simulink model "Trayectoria"  (R2023b)
settings: Solver=ode8  StartTime=0.0  StopTime=t6  FixedStep=0.01  RelTol=1e-3
undefined symbols (not defined in the file): alpha8, cL, cO, cpL, cpO, cpS, cS, gammaO, gammaS, k1, k2, k3, k4, klL, klO, klS, muO, muS, r8, t3, xr8, xrLB, xrLH, xrLPA, xrLR, xrLSA, xrLTA, xrO, xrS
libraries: vrlib x1
settings Model: Creator=olegalexandrocraviotog.  LastModifiedBy=olegalexandrocraviotog.

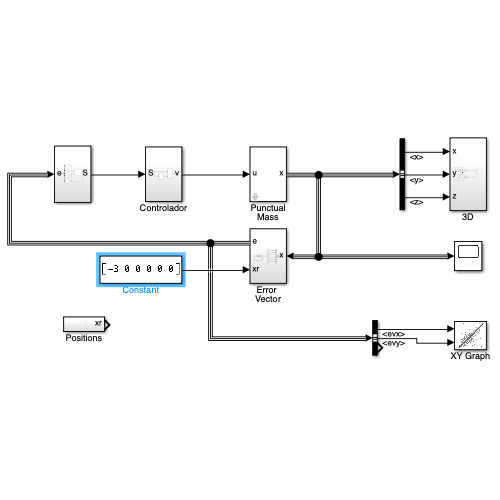
[thumbnail: Simulink's stored preview of the top-level diagram]
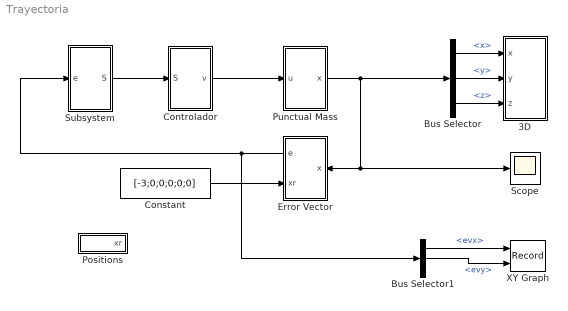
== system Trayectoria ==
  3D : Subsystem
  Bus Selector : BusSelector  OutputSignals=x,y,z
  Bus Selector1 : BusSelector  OutputSignals=evx,evy,evz
  Constant : Constant  Value=[-3;0;0;0;0;0]
  Controlador : Subsystem
  Error Vector : Subsystem
      settings: PortSchema="{\"entries\":[{\"content\":{\"sides\":[{\"content\":{\"connectorIds\":[\"Out1\",\"In1\"]},\"type\":\"ConnectorPlacement.EquallySpacedRectSide\",\"uuid\":\"f657f758-fbd3-4a41-9063-d27a9332990f\"},{\"content\":{\"connectorIds\":[\"In2\"],\"side\":\"RIGHT\"},\"type\":\"ConnectorPlacement.EquallySpacedRectSide\",\"uuid\":\"1c515ff8-89aa-408f-b30d-a9af781c1d92\"},{\"content\":{\"side\":\"TOP\"},\"type\":\"ConnectorPlacement.EquallySpacedRectSide\",\"uuid\":\"e6b04dad-d129-4308-a4a4-85eae89abd10\"}]},\"type\":\"ConnectorPlacement.EquallySpacedConnector\",\"uuid\":\"97b78294-1485-42d0-98d9-31abf3c44744\"}],\"packageUris\":[\"http://schema.mathworks.com/mf0/Connector/R2020b\"],\"version\":\"1.0\"}"
  Positions : Subsystem
  Punctual Mass : Subsystem  mask{A=[0 0 0 1 0 0; 0 0 0 0 1 0; 0 0 0 0 0 1; 0 0 0 0 0 0; 0 0 0 0 0 0; 0 0 0 0 0 0], B=[0 0 0; 0 0 0; 0 0 0; 1 0 0; 0 1 0; 0 0 1]}
  Scope : Scope
  Subsystem : Subsystem
  XY Graph : Record  FileSettingsInternal="{\"entries\":[{\"content\":{\"excelSettings\":{\"content\":{},\"type\":\"Streamout.ExcelSettings\"}},\"type\":\"Streamout.FileSettingStorage\",\"uuid\":\"\"}],\"packageUris\":[\"http:\\/\\/schema.mathworks.com\\/mf0\\/streamout_blocks\\/R2020a\"],\"version\":\"1.0\"}"  Layout=[1 1]  SignalsInternal="{\"entries\":[{\"content\":{\"signals\":[{\"content\":{\"blockPath\":[],\"dimensions\":[1],\"domain\":\"\",\"lineColor\":\"#a2142f\",\"plots\":[1],\"port\":1,\"sid\":[\"\"],\"signalID\":12236,\"signalName\":\"<evx>\"},\"type\":\"RecordBlkView.Signal\",\"uuid\":\"\"},{\"content\":{\"blockPath\":[],\"dimensions\":[1],\"domain\":\"\",\"lineColor\":\"#139fff\",\"plots\":[1],\"port\":2,\"sid\":[\"\"],\"signalID\":12240,\"signalName\":\"<evy>\"},\"type\":\"RecordBlkView.Signal\",\"uuid\":\"\"}]},\"type\":\"RecordBlkView.InputSignals\",\"uuid\":\"\"}],\"packageUris\":[\"http:\\/\\/schema.mathworks.com\\/mf0\\/streamout_blocks\\/R2020a\"],\"version\":\"1.0\"}"  VisualizationBindings="{\"xyplotplugin\":{\"info\":[{\"series\":[{\"bindingParametersList\":[{\"parameter\":\"X-Axis\",\"signalID\":12236,\"signalName\":\"<evx>\"},{\"parameter\":\"Y-Axis\",\"signalID\":12240,\"signalName\":\"<evy>\"}],\"seriesID\":43551}],\"subplotID\":1}]}}"  CompatibilityTag=XY
  wires:
  Punctual Mass/1(x) -> Scope/1, Error Vector/2(x), Bus Selector/1
  Bus Selector/1 -> 3D/1(x)  "<x>"
  Bus Selector/2 -> 3D/2(y)  "<y>"
  Bus Selector/3 -> 3D/3(z)  "<z>"
  Controlador/1(v) -> Punctual Mass/1(u)
  Subsystem/1(S) -> Controlador/1(S)
  Error Vector/1(e) -> Subsystem/1(e), Bus Selector1/1
  Bus Selector1/1 -> XY Graph/1  "<evx>"
  Constant/1 -> Error Vector/1(xr)
  Bus Selector1/2 -> XY Graph/2  "<evy>"

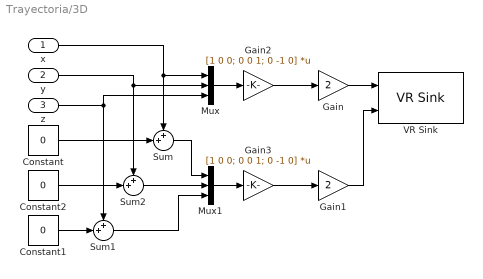
== system Trayectoria/3D ==
  x : Inport
  y : Inport  Port=2
  z : Inport  Port=3
  Constant : Constant  Value=0
  Constant1 : Constant  Value=0
  Constant2 : Constant  Value=0
  Gain : Gain  Gain=2
  Gain1 : Gain  Gain=2
  Gain2 : Gain  Gain=[1 0 0; 0 0 1; 0 -1 0]  Multiplication=Matrix(K*u)
  Gain3 : Gain  Gain=[1 0 0; 0 0 1; 0 -1 0]  Multiplication=Matrix(K*u)
  Mux : Mux  Inputs=3
  Mux1 : Mux  Inputs=3
  Sum : Sum  Inputs=++|
  Sum1 : Sum  Inputs=++|
  Sum2 : Sum  Inputs=++|
  VR Sink : vrlib/VR Sink  InstantiateOnLoad=on  SampleTime=0.01  ViewEnable=on  RemoteChange=off  RemoteView=off  FieldsWritten=Masa.translation.3.1.1.double#Pelota.position.3.1.1.double  WorldFileName=/Users/olegalexandrocraviotog./Documents/MATLAB/MasaPuntual/Imagenes3D/Trayectoria3D.x3d  AutoView=off  VideoDimensions=[]  AllowVariableSize=off
  wires:
  z/1 -> Sum1/1, Mux/3
  y/1 -> Sum2/1, Mux/2
  x/1 -> Mux/1, Sum/1
  Gain2/1 -> Gain/1
  Mux/1 -> Gain2/1
  Sum1/1 -> Mux1/3
  Sum2/1 -> Mux1/2
  Sum/1 -> Mux1/1
  Gain3/1 -> Gain1/1
  Constant2/1 -> Sum2/2
  Constant1/1 -> Sum1/2
  Gain1/1 -> VR Sink/2
  Constant/1 -> Sum/2
  Mux1/1 -> Gain3/1
  Gain/1 -> VR Sink/1

== system Trayectoria/Controlador ==
  S : Inport
  Subsystem1 : Subsystem
  Subsystem2 : Subsystem
  v : Outport
  wires:
  S/1 -> Subsystem2/1(S), Subsystem1/1(S)
  Subsystem2/1(dZ) -> Subsystem1/2(dZ)
  Subsystem1/1(v) -> v/1

== system Trayectoria/Error Vector ==
  xr : Inport
  x : Inport  Port=2
  Bus Creator : BusCreator  Inputs=6
  Demux : Demux  Outputs=6
  Sum : Sum  Inputs=|+-
  e : Outport
  wires:
  x/1 -> Sum/1
  xr/1 -> Sum/2
  Bus Creator/1 -> e/1
  Sum/1 -> Demux/1
  Demux/1 -> Bus Creator/1  "ex"
  Demux/2 -> Bus Creator/2  "ey"
  Demux/3 -> Bus Creator/3  "ez"
  Demux/4 -> Bus Creator/4  "evx"
  Demux/5 -> Bus Creator/5  "evy"
  Demux/6 -> Bus Creator/6  "evz"

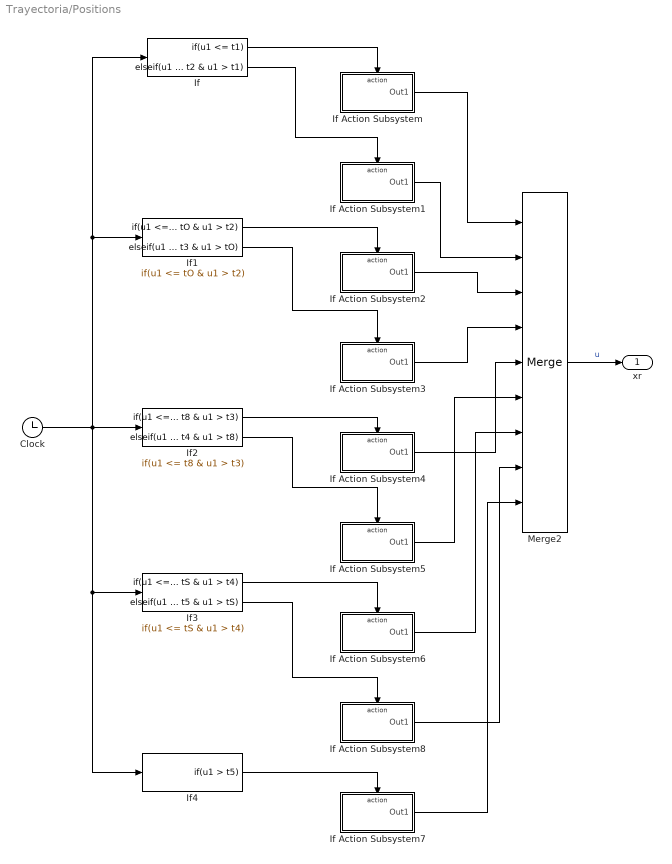
== system Trayectoria/Positions ==
  Clock : Clock
  If : If  IfExpression=u1 <= t1  ElseIfExpressions=u1 <= t2 & u1 > t1  ShowElse=off
  If Action Subsystem : Subsystem  TreatAsAtomicUnit=on
  If Action Subsystem1 : Subsystem  TreatAsAtomicUnit=on
  If Action Subsystem2 : Subsystem  TreatAsAtomicUnit=on
  If Action Subsystem3 : Subsystem  TreatAsAtomicUnit=on
  If Action Subsystem4 : Subsystem  TreatAsAtomicUnit=on
  If Action Subsystem5 : Subsystem  TreatAsAtomicUnit=on
  If Action Subsystem6 : Subsystem  TreatAsAtomicUnit=on
  If Action Subsystem7 : Subsystem  TreatAsAtomicUnit=on
  If Action Subsystem8 : Subsystem  TreatAsAtomicUnit=on
  If1 : If  IfExpression=u1 <= tO & u1 > t2  ElseIfExpressions=u1 <= t3 & u1 > tO  ShowElse=off
  If2 : If  IfExpression=u1 <= t8 & u1 > t3  ElseIfExpressions=u1 <= t4 & u1 > t8  ShowElse=off
  If3 : If  IfExpression=u1 <= tS & u1 > t4  ElseIfExpressions=u1 <= t5 & u1 > tS  ShowElse=off
  If4 : If  IfExpression=u1 > t5  ShowElse=off
  Merge2 : Merge  Inputs=9
  xr : Outport
  wires:
  If/1 -> If Action Subsystem/Action
  Clock/1 -> If3/1, If4/1, If2/1, If1/1, If/1
  Merge2/1 -> xr/1  "u"
  If Action Subsystem/1(Out1) -> Merge2/1
  If Action Subsystem1/1(Out1) -> Merge2/2
  If Action Subsystem2/1(Out1) -> Merge2/3
  If Action Subsystem3/1(Out1) -> Merge2/4
  If Action Subsystem4/1(Out1) -> Merge2/5
  If Action Subsystem5/1(Out1) -> Merge2/6
  If Action Subsystem6/1(Out1) -> Merge2/7
  If Action Subsystem8/1(Out1) -> Merge2/8
  If Action Subsystem7/1(Out1) -> Merge2/9
  If/2 -> If Action Subsystem1/Action
  If1/1 -> If Action Subsystem2/Action
  If1/2 -> If Action Subsystem3/Action
  If2/1 -> If Action Subsystem4/Action
  If2/2 -> If Action Subsystem5/Action
  If3/1 -> If Action Subsystem6/Action
  If3/2 -> If Action Subsystem8/Action
  If4/1 -> If Action Subsystem7/Action

== system Trayectoria/Punctual Mass ==
  u : Inport
  Bus Creator : BusCreator  Inputs=6
  Constant : Constant  Value=[0;0;0]
  Demux : Demux  Outputs=6
  Gain : Gain  Gain=A  Multiplication=Matrix(K*u)
  Gain1 : Gain  Gain=B  Multiplication=Matrix(K*u)
  Integrator : Integrator  InitialCondition=[0;0;0;0;0;0]
  Sum : Sum  Inputs=|++
  Sum1 : Sum  Inputs=++|
  x : Outport
  wires:
  u/1 -> Sum1/2
  Sum1/1 -> Gain1/1
  Constant/1 -> Sum1/1
  Gain1/1 -> Sum/1
  Integrator/1 -> Gain/1, Demux/1
  Sum/1 -> Integrator/1
  Gain/1 -> Sum/2
  Demux/3 -> Bus Creator/3  "z"
  Demux/1 -> Bus Creator/1  "x"
  Demux/2 -> Bus Creator/2  "y"
  Demux/4 -> Bus Creator/4  "vx"
  Demux/5 -> Bus Creator/5  "vy"
  Demux/6 -> Bus Creator/6  "vz"
  Bus Creator/1 -> x/1

== system Trayectoria/Subsystem ==
  e : Inport
  Descendent Spiral : Subsystem
  Eight on a Sphere : Subsystem
  Looping : Subsystem
  Positions : Subsystem
  Staight Line : Subsystem
  S : Outport
  wires:
  e/1 -> Looping/1(e), Staight Line/1(e), Descendent Spiral/1(e), Eight on a Sphere/1(e)
  Staight Line/1(Sj) -> Positions/1(Straight Line)
  Eight on a Sphere/1(S4) -> Positions/3(Egith on a Sphere)
  Descendent Spiral/1(S6) -> Positions/4(Descending Spiral), S/1
  Looping/1(S6) -> Positions/2(Looping)

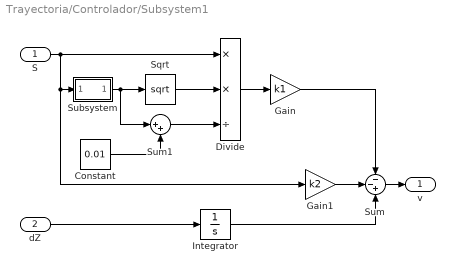
== system Trayectoria/Controlador/Subsystem1 ==
  S : Inport
  dZ : Inport  Port=2
  Constant : Constant  Value=0.01
  Divide : Product  Inputs=**/
  Gain : Gain  Gain=k1
  Gain1 : Gain  Gain=k2
  Integrator : Integrator
  Sqrt : Sqrt
  Subsystem : Subsystem
      mask Display: disp('||  ||');
  Sum : Sum  Inputs=--+
  Sum1 : Sum  Inputs=|++
  v : Outport
  wires:
  dZ/1 -> Integrator/1
  Divide/1 -> Gain/1
  Sum1/1 -> Divide/3
  Sum/1 -> v/1
  Integrator/1 -> Sum/3
  S/1 -> Gain1/1, Subsystem/1(In1), Divide/1
  Subsystem/1(Out1) -> Sum1/1, Sqrt/1
  Constant/1 -> Sum1/2
  Gain1/1 -> Sum/2
  Sqrt/1 -> Divide/2
  Gain/1 -> Sum/1

== system Trayectoria/Controlador/Subsystem2 ==
  S : Inport
  Constant : Constant  Value=0.01
  Gain2 : Gain  Gain=k3
  Gain3 : Gain  Gain=k4
  Product : Product  Inputs=*/
  Subsystem : Subsystem
      mask Display: disp('||  ||');
  Sum : Sum  Inputs=|++
  Sum1 : Sum  Inputs=--
  dZ : Outport
  wires:
  Sum1/1 -> dZ/1
  Subsystem/1(Out1) -> Sum/1
  Product/1 -> Gain2/1
  Gain3/1 -> Sum1/2
  Sum/1 -> Product/2
  Constant/1 -> Sum/2
  Gain2/1 -> Sum1/1
  S/1 -> Product/1, Gain3/1, Subsystem/1(In1)

== system Trayectoria/Positions/If Action Subsystem ==
  Action Port : ActionPort  ActionPortLabel=if(u1 <= t1)
  Constant : Constant  Value=xrLH
  Out1 : Outport
  wires:
  Constant/1 -> Out1/1

== system Trayectoria/Positions/If Action Subsystem1 ==
  Action Port : ActionPort  ActionPortLabel=elseif(u1 <= t2 & u1 > t1)
  Constant : Constant  Value=xrLPA
  Out1 : Outport
  wires:
  Constant/1 -> Out1/1

== system Trayectoria/Positions/If Action Subsystem2 ==
  Action Port : ActionPort  ActionPortLabel=if(u1 <= tO & u1 > t2)
  Constant : Constant  Value=xrO
  Out1 : Outport
  wires:
  Constant/1 -> Out1/1

== system Trayectoria/Positions/If Action Subsystem3 ==
  Action Port : ActionPort  ActionPortLabel=elseif(u1 <= t3 & u1 > tO)
  Constant : Constant  Value=xrLSA
  Out1 : Outport
  wires:
  Constant/1 -> Out1/1

== system Trayectoria/Positions/If Action Subsystem4 ==
  Action Port : ActionPort  ActionPortLabel=if(u1 <= t8 & u1 > t3)
  Constant : Constant  Value=xr8
  Out1 : Outport
  wires:
  Constant/1 -> Out1/1

== system Trayectoria/Positions/If Action Subsystem5 ==
  Action Port : ActionPort  ActionPortLabel=elseif(u1 <= t4 & u1 > t8)
  Constant : Constant  Value=xrLTA
  Out1 : Outport
  wires:
  Constant/1 -> Out1/1

== system Trayectoria/Positions/If Action Subsystem6 ==
  Action Port : ActionPort  ActionPortLabel=if(u1 <= tS & u1 > t4)
  Constant : Constant  Value=xrS
  Out1 : Outport
  wires:
  Constant/1 -> Out1/1

== system Trayectoria/Positions/If Action Subsystem7 ==
  Action Port : ActionPort  ActionPortLabel=if(u1 > t5)
  Constant : Constant  Value=xrLB
  Out1 : Outport
  wires:
  Constant/1 -> Out1/1

== system Trayectoria/Positions/If Action Subsystem8 ==
  Action Port : ActionPort  ActionPortLabel=elseif(u1 <= t5 & u1 > tS)
  Constant : Constant  Value=xrLR
  Out1 : Outport
  wires:
  Constant/1 -> Out1/1

== system Trayectoria/Subsystem/Descendent Spiral ==
  e : Inport
  Bus Selector3 : BusSelector  OutputSignals=ez,evz
  Mux : Mux  Inputs=3
  Subsystem : Subsystem  mask{mu=muS, gama=gammaS}
      mask prompts: gama "gamma"
  Subsystem1 : Subsystem  mask{mu=muS, gama=gammaS}
      mask prompts: gama "gamma"
  Subsystem2 : Subsystem  mask{k=klS, c=cS, cp=cpS}
  S6 : Outport
  wires:
  Mux/1 -> S6/1
  Subsystem2/1(Sz) -> Mux/3
  Bus Selector3/2 -> Subsystem2/2(ev)  "<evz>"
  Bus Selector3/1 -> Subsystem2/1(e)  "<ez>"
  e/1 -> Subsystem1/1(e), Subsystem/1(e), Bus Selector3/1
  Subsystem1/1(Sy) -> Mux/2
  Subsystem/1(Sx) -> Mux/1

== system Trayectoria/Subsystem/Eight on a Sphere ==
  e : Inport
  Mux : Mux  Inputs=3
  Subsystem : Subsystem  mask{apha=alpha8, r=r8}
      mask prompts: apha "alpha"
  Subsystem1 : Subsystem  mask{apha=alpha8, r=r8}
      mask prompts: apha "alpha"
  Subsystem2 : Subsystem  mask{apha=alpha8, r=r8}
      mask prompts: apha "alpha"
  S4 : Outport
  wires:
  e/1 -> Subsystem2/1(e), Subsystem/1(e), Subsystem1/1(e)
  Subsystem1/1(Sy) -> Mux/2
  Subsystem/1(Sx) -> Mux/1
  Subsystem2/1(Sz) -> Mux/3
  Mux/1 -> S4/1

== system Trayectoria/Subsystem/Looping ==
  e : Inport
  Bus Selector3 : BusSelector  OutputSignals=ey,evy
  Mux : Mux  Inputs=3
  Subsystem : Subsystem  mask{mu=muO, gama=gammaO}
      mask prompts: gama "gamma"
  Subsystem1 : Subsystem  mask{mu=muO, gama=gammaO}
      mask prompts: gama "gamma"
  Subsystem2 : Subsystem  mask{k=klO, c=cO, cp=cpO}
  S6 : Outport
  wires:
  Subsystem/1(Sx) -> Mux/1
  e/1 -> Bus Selector3/1, Subsystem/1(e), Subsystem1/1(e)
  Bus Selector3/1 -> Subsystem2/1(e)  "<ey>"
  Bus Selector3/2 -> Subsystem2/2(ev)  "<evy>"
  Mux/1 -> S6/1
  Subsystem2/1(Sy) -> Mux/2
  Subsystem1/1(Sz) -> Mux/3

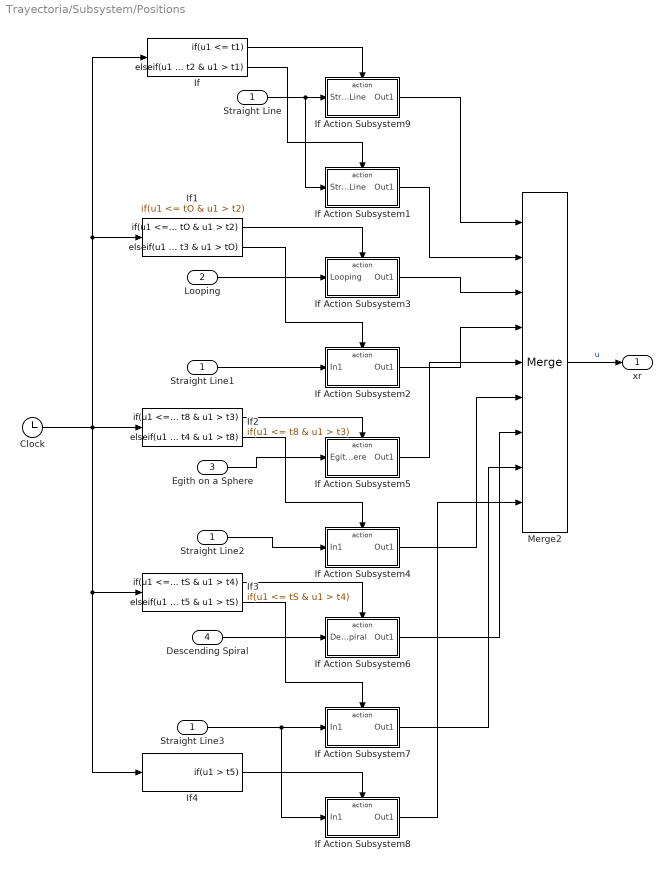
== system Trayectoria/Subsystem/Positions ==
  Straight Line : Inport
  Looping : Inport  Port=2
  Egith on a Sphere : Inport  Port=3
  Descending Spiral : Inport  Port=4
  Clock : Clock
  If : If  IfExpression=u1 <= t1  ElseIfExpressions=u1 <= t2 & u1 > t1  ShowElse=off
  If Action Subsystem1 : Subsystem  TreatAsAtomicUnit=on
  If Action Subsystem2 : Subsystem  TreatAsAtomicUnit=on
  If Action Subsystem3 : Subsystem  TreatAsAtomicUnit=on
  If Action Subsystem4 : Subsystem  TreatAsAtomicUnit=on
  If Action Subsystem5 : Subsystem  TreatAsAtomicUnit=on
  If Action Subsystem6 : Subsystem  TreatAsAtomicUnit=on
  If Action Subsystem7 : Subsystem  TreatAsAtomicUnit=on
  If Action Subsystem8 : Subsystem  TreatAsAtomicUnit=on
  If Action Subsystem9 : Subsystem  TreatAsAtomicUnit=on
  If1 : If  IfExpression=u1 <= tO & u1 > t2  ElseIfExpressions=u1 <= t3 & u1 > tO  ShowElse=off
  If2 : If  IfExpression=u1 <= t8 & u1 > t3  ElseIfExpressions=u1 <= t4 & u1 > t8  ShowElse=off
  If3 : If  IfExpression=u1 <= tS & u1 > t4  ElseIfExpressions=u1 <= t5 & u1 > tS  ShowElse=off
  If4 : If  IfExpression=u1 > t5  ShowElse=off
  Merge2 : Merge  Inputs=9
  Straight Line1 : InportShadow
  Straight Line2 : InportShadow
  Straight Line3 : InportShadow
  xr : Outport
  wires:
  Clock/1 -> If3/1, If4/1, If2/1, If1/1, If/1
  Merge2/1 -> xr/1  "u"
  If/1 -> If Action Subsystem9/Action
  If/2 -> If Action Subsystem1/Action
  If1/1 -> If Action Subsystem3/Action
  If1/2 -> If Action Subsystem2/Action
  If2/1 -> If Action Subsystem5/Action
  If2/2 -> If Action Subsystem4/Action
  If3/1 -> If Action Subsystem6/Action
  If3/2 -> If Action Subsystem7/Action
  If4/1 -> If Action Subsystem8/Action
  Straight Line/1 -> If Action Subsystem1/1(Straight Line), If Action Subsystem9/1(Straight Line)
  Looping/1 -> If Action Subsystem3/1(Looping)
  Straight Line1/1 -> If Action Subsystem2/1(In1)
  Egith on a Sphere/1 -> If Action Subsystem5/1(Egith on a Sphere)
  Straight Line2/1 -> If Action Subsystem4/1(In1)
  Descending Spiral/1 -> If Action Subsystem6/1(Descending Spiral)
  Straight Line3/1 -> If Action Subsystem8/1(In1), If Action Subsystem7/1(In1)
  If Action Subsystem9/1(Out1) -> Merge2/1
  If Action Subsystem1/1(Out1) -> Merge2/2
  If Action Subsystem3/1(Out1) -> Merge2/3
  If Action Subsystem2/1(Out1) -> Merge2/4
  If Action Subsystem5/1(Out1) -> Merge2/5
  If Action Subsystem4/1(Out1) -> Merge2/6
  If Action Subsystem6/1(Out1) -> Merge2/7
  If Action Subsystem7/1(Out1) -> Merge2/8
  If Action Subsystem8/1(Out1) -> Merge2/9

== system Trayectoria/Subsystem/Staight Line ==
  e : Inport
  Bus Selector1 : BusSelector  OutputSignals=ex,evx
  Bus Selector2 : BusSelector  OutputSignals=ey,evy
  Bus Selector3 : BusSelector  OutputSignals=ez,evz
  Mux : Mux  Inputs=3
  Subsystem : Subsystem  mask{k=klL(1), c=cL(1), cp=cpL(1)}
  Subsystem1 : Subsystem  mask{k=klL(2), c=cL(2), cp=cpL(2)}
  Subsystem2 : Subsystem  mask{k=klL(3), c=cL(3), cp=cpL(3)}
  Sj : Outport
  wires:
  e/1 -> Bus Selector1/1, Bus Selector3/1, Bus Selector2/1
  Bus Selector1/1 -> Subsystem/1(e)  "<ex>"
  Bus Selector1/2 -> Subsystem/2(ev)  "<evx>"
  Bus Selector2/1 -> Subsystem1/1(e)  "<ey>"
  Bus Selector2/2 -> Subsystem1/2(ev)  "<evy>"
  Bus Selector3/1 -> Subsystem2/1(e)  "<ez>"
  Bus Selector3/2 -> Subsystem2/2(ev)  "<evz>"
  Subsystem1/1(Sy) -> Mux/2
  Subsystem/1(Sx) -> Mux/1
  Subsystem2/1(Sz) -> Mux/3
  Mux/1 -> Sj/1

== system Trayectoria/Controlador/Subsystem1/Subsystem ==
  In1 : Inport
  Dot Product : DotProduct  OutDataTypeStr=Inherit: Inherit via internal rule
  Sqrt : Sqrt
  Out1 : Outport
  wires:
  Dot Product/1 -> Sqrt/1
  Sqrt/1 -> Out1/1
  In1/1 -> Dot Product/2, Dot Product/1

== system Trayectoria/Controlador/Subsystem2/Subsystem ==
  In1 : Inport
  Dot Product : DotProduct  OutDataTypeStr=Inherit: Inherit via internal rule
  Sqrt : Sqrt
  Out1 : Outport
  wires:
  Dot Product/1 -> Sqrt/1
  Sqrt/1 -> Out1/1
  In1/1 -> Dot Product/2, Dot Product/1

== system Trayectoria/Subsystem/Descendent Spiral/Subsystem ==
  e : Inport
  Bus Selector1 : BusSelector  OutputSignals=evx,ex,ey
  Gain : Gain  Gain=mu
  Gain1 : Gain  Gain=gama
  Math Function : Math  Operator=square
  Math Function1 : Math  Operator=square
  Product : Product
  Sum : Sum
  Sum1 : Sum  Inputs=+--+
  Sx : Outport
  wires:
  e/1 -> Bus Selector1/1
  Math Function/1 -> Sum/1
  Math Function1/1 -> Sum/2
  Bus Selector1/3 -> Math Function1/1, Gain1/1  "<ey>"
  Bus Selector1/2 -> Product/1, Math Function/1, Gain/1  "<ex>"
  Bus Selector1/1 -> Sum1/1  "<evx>"
  Gain/1 -> Sum1/2
  Gain1/1 -> Sum1/3
  Sum/1 -> Product/2
  Product/1 -> Sum1/4
  Sum1/1 -> Sx/1

== system Trayectoria/Subsystem/Descendent Spiral/Subsystem1 ==
  e : Inport
  Bus Selector1 : BusSelector  OutputSignals=evy,ey,ex
  Gain : Gain  Gain=mu
  Gain1 : Gain  Gain=gama
  Math Function : Math  Operator=square
  Math Function1 : Math  Operator=square
  Product : Product
  Sum : Sum
  Sum1 : Sum  Inputs=+-++
  Sy : Outport
  wires:
  Sum1/1 -> Sy/1
  Math Function1/1 -> Sum/2
  Math Function/1 -> Sum/1
  e/1 -> Bus Selector1/1
  Bus Selector1/2 -> Product/1, Math Function/1, Gain/1  "<ey>"
  Bus Selector1/3 -> Math Function1/1, Gain1/1  "<ex>"
  Sum/1 -> Product/2
  Bus Selector1/1 -> Sum1/1  "<evy>"
  Gain/1 -> Sum1/2
  Gain1/1 -> Sum1/3
  Product/1 -> Sum1/4

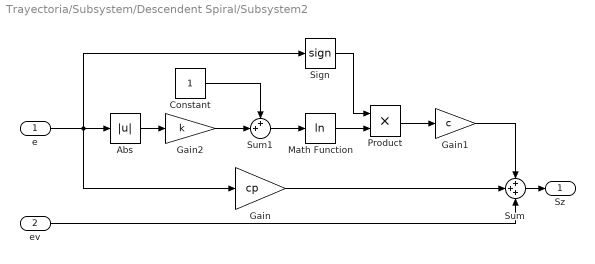
== system Trayectoria/Subsystem/Descendent Spiral/Subsystem2 ==
  e : Inport
  ev : Inport  Port=2
  Abs : Abs  SaturateOnIntegerOverflow=off
  Constant : Constant
  Gain : Gain  Gain=cp
  Gain1 : Gain  Gain=c
  Gain2 : Gain  Gain=k
  Math Function : Math  Operator=log
  Product : Product
  Sign : Signum
  Sum : Sum  Inputs=+++
  Sum1 : Sum  Inputs=++|
  Sz : Outport
  wires:
  Gain/1 -> Sum/2
  Constant/1 -> Sum1/1
  Abs/1 -> Gain2/1
  Product/1 -> Gain1/1
  Sum1/1 -> Math Function/1
  ev/1 -> Sum/3
  Sum/1 -> Sz/1
  Math Function/1 -> Product/2
  e/1 -> Abs/1, Sign/1, Gain/1
  Gain1/1 -> Sum/1
  Sign/1 -> Product/1
  Gain2/1 -> Sum1/2

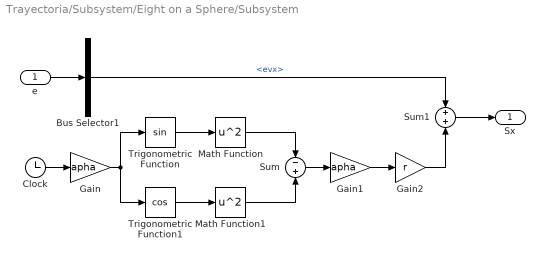
== system Trayectoria/Subsystem/Eight on a Sphere/Subsystem ==
  e : Inport
  Bus Selector1 : BusSelector  OutputSignals=evx
  Clock : Clock
  Gain : Gain  Gain=apha
  Gain1 : Gain  Gain=apha
  Gain2 : Gain  Gain=r
  Math Function1 : Math  Operator=square
  Math Function : Math  Operator=square
  Sum : Sum  Inputs=-+
  Sum1 : Sum
  Trigonometric Function : Trigonometry
  Trigonometric Function1 : Trigonometry  Operator=cos
  Sx : Outport
  wires:
  e/1 -> Bus Selector1/1
  Trigonometric Function/1 -> Math Function/1
  Trigonometric Function1/1 -> Math Function1/1
  Math Function/1 -> Sum/1
  Math Function1/1 -> Sum/2
  Gain/1 -> Trigonometric Function/1, Trigonometric Function1/1
  Clock/1 -> Gain/1
  Sum/1 -> Gain1/1
  Gain1/1 -> Gain2/1
  Gain2/1 -> Sum1/2
  Bus Selector1/1 -> Sum1/1  "<evx>"
  Sum1/1 -> Sx/1

== system Trayectoria/Subsystem/Eight on a Sphere/Subsystem1 ==
  e : Inport
  Bus Selector : BusSelector  OutputSignals=evy
  Clock : Clock
  Constant : Constant  Value=t3
  Gain2 : Gain  Gain=apha
  Gain3 : Gain  Gain=apha
  Gain4 : Gain  Gain=r
  Sum1 : Sum  Inputs=|+-
  Sum2 : Sum  Inputs=|+-
  Trigonometric Function : Trigonometry  Operator=cos
  Sy : Outport
  wires:
  e/1 -> Bus Selector/1
  Bus Selector/1 -> Sum1/1  "<evy>"
  Trigonometric Function/1 -> Gain3/1
  Sum1/1 -> Sy/1
  Gain4/1 -> Sum1/2
  Gain2/1 -> Trigonometric Function/1
  Gain3/1 -> Gain4/1
  Sum2/1 -> Gain2/1
  Clock/1 -> Sum2/1
  Constant/1 -> Sum2/2

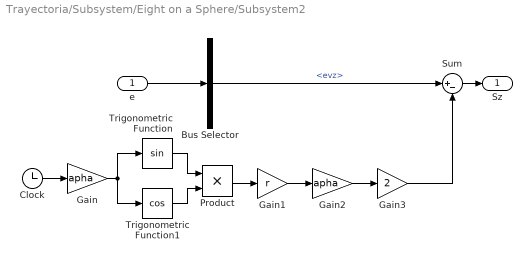
== system Trayectoria/Subsystem/Eight on a Sphere/Subsystem2 ==
  e : Inport
  Bus Selector : BusSelector  OutputSignals=evz
  Clock : Clock
  Gain : Gain  Gain=apha
  Gain1 : Gain  Gain=r
  Gain2 : Gain  Gain=apha
  Gain3 : Gain  Gain=2
  Product : Product
  Sum : Sum  Inputs=|+-
  Trigonometric Function : Trigonometry
  Trigonometric Function1 : Trigonometry  Operator=cos
  Sz : Outport
  wires:
  Sum/1 -> Sz/1
  Bus Selector/1 -> Sum/1  "<evz>"
  e/1 -> Bus Selector/1
  Trigonometric Function/1 -> Product/1
  Trigonometric Function1/1 -> Product/2
  Gain/1 -> Trigonometric Function/1, Trigonometric Function1/1
  Clock/1 -> Gain/1
  Product/1 -> Gain1/1
  Gain1/1 -> Gain2/1
  Gain2/1 -> Gain3/1
  Gain3/1 -> Sum/2

== system Trayectoria/Subsystem/Looping/Subsystem ==
  e : Inport
  Bus Selector1 : BusSelector  OutputSignals=evx,ex,ez
  Gain : Gain  Gain=mu
  Gain1 : Gain  Gain=gama
  Math Function : Math  Operator=square
  Math Function1 : Math  Operator=square
  Product : Product
  Sum : Sum
  Sum1 : Sum  Inputs=+--+
  Sx : Outport
  wires:
  Sum1/1 -> Sx/1
  Product/1 -> Sum1/4
  Sum/1 -> Product/2
  Gain1/1 -> Sum1/3
  Gain/1 -> Sum1/2
  Math Function1/1 -> Sum/2
  Math Function/1 -> Sum/1
  e/1 -> Bus Selector1/1
  Bus Selector1/1 -> Sum1/1  "<evx>"
  Bus Selector1/2 -> Product/1, Math Function/1, Gain/1  "<ex>"
  Bus Selector1/3 -> Math Function1/1, Gain1/1  "<ez>"

== system Trayectoria/Subsystem/Looping/Subsystem1 ==
  e : Inport
  Bus Selector1 : BusSelector  OutputSignals=evz,ez,ex
  Gain : Gain  Gain=mu
  Gain1 : Gain  Gain=gama
  Math Function : Math  Operator=square
  Math Function1 : Math  Operator=square
  Product : Product
  Sum : Sum
  Sum1 : Sum  Inputs=+-++
  Sz : Outport
  wires:
  Product/1 -> Sum1/4
  Gain1/1 -> Sum1/3
  Gain/1 -> Sum1/2
  Sum/1 -> Product/2
  e/1 -> Bus Selector1/1
  Math Function/1 -> Sum/1
  Math Function1/1 -> Sum/2
  Sum1/1 -> Sz/1
  Bus Selector1/1 -> Sum1/1  "<evz>"
  Bus Selector1/2 -> Gain/1, Product/1, Math Function/1  "<ez>"
  Bus Selector1/3 -> Math Function1/1, Gain1/1  "<ex>"

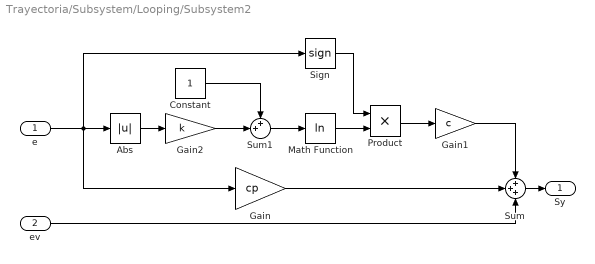
== system Trayectoria/Subsystem/Looping/Subsystem2 ==
  e : Inport
  ev : Inport  Port=2
  Abs : Abs  SaturateOnIntegerOverflow=off
  Constant : Constant
  Gain : Gain  Gain=cp
  Gain1 : Gain  Gain=c
  Gain2 : Gain  Gain=k
  Math Function : Math  Operator=log
  Product : Product
  Sign : Signum
  Sum : Sum  Inputs=+++
  Sum1 : Sum  Inputs=++|
  Sy : Outport
  wires:
  Gain2/1 -> Sum1/2
  Sign/1 -> Product/1
  Gain1/1 -> Sum/1
  e/1 -> Gain/1, Sign/1, Abs/1
  Math Function/1 -> Product/2
  Sum/1 -> Sy/1
  ev/1 -> Sum/3
  Sum1/1 -> Math Function/1
  Product/1 -> Gain1/1
  Abs/1 -> Gain2/1
  Constant/1 -> Sum1/1
  Gain/1 -> Sum/2

== system Trayectoria/Subsystem/Positions/If Action Subsystem1 ==
  Straight Line : Inport
  Action Port : ActionPort  ActionPortLabel=elseif(u1 <= t2 & u1 > t1)
  Out1 : Outport
  wires:
  Straight Line/1 -> Out1/1

== system Trayectoria/Subsystem/Positions/If Action Subsystem2 ==
  In1 : Inport
  Action Port : ActionPort  ActionPortLabel=elseif(u1 <= t3 & u1 > tO)
  Out1 : Outport
  wires:
  In1/1 -> Out1/1

== system Trayectoria/Subsystem/Positions/If Action Subsystem3 ==
  Looping : Inport
  Action Port : ActionPort  ActionPortLabel=if(u1 <= tO & u1 > t2)
  Out1 : Outport
  wires:
  Looping/1 -> Out1/1

== system Trayectoria/Subsystem/Positions/If Action Subsystem4 ==
  In1 : Inport
  Action Port : ActionPort  ActionPortLabel=elseif(u1 <= t4 & u1 > t8)
  Out1 : Outport
  wires:
  In1/1 -> Out1/1

== system Trayectoria/Subsystem/Positions/If Action Subsystem5 ==
  Egith on a Sphere : Inport
  Action Port : ActionPort  ActionPortLabel=if(u1 <= t8 & u1 > t3)
  Out1 : Outport
  wires:
  Egith on a Sphere/1 -> Out1/1

== system Trayectoria/Subsystem/Positions/If Action Subsystem6 ==
  Descending Spiral : Inport
  Action Port : ActionPort  ActionPortLabel=if(u1 <= tS & u1 > t4)
  Out1 : Outport
  wires:
  Descending Spiral/1 -> Out1/1

== system Trayectoria/Subsystem/Positions/If Action Subsystem7 ==
  In1 : Inport
  Action Port : ActionPort  ActionPortLabel=elseif(u1 <= t5 & u1 > tS)
  Out1 : Outport
  wires:
  In1/1 -> Out1/1

== system Trayectoria/Subsystem/Positions/If Action Subsystem8 ==
  In1 : Inport
  Action Port : ActionPort  ActionPortLabel=if(u1 > t5)
  Out1 : Outport
  wires:
  In1/1 -> Out1/1

== system Trayectoria/Subsystem/Positions/If Action Subsystem9 ==
  Straight Line : Inport
  Action Port : ActionPort  ActionPortLabel=if(u1 <= t1)
  Out1 : Outport
  wires:
  Straight Line/1 -> Out1/1

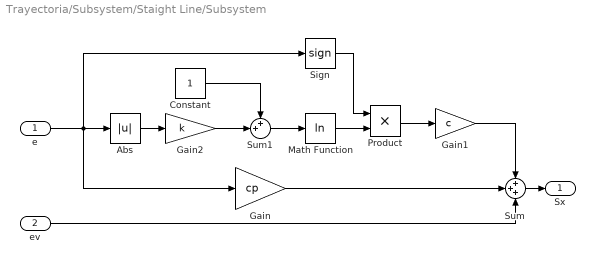
== system Trayectoria/Subsystem/Staight Line/Subsystem ==
  e : Inport
  ev : Inport  Port=2
  Abs : Abs  SaturateOnIntegerOverflow=off
  Constant : Constant
  Gain : Gain  Gain=cp
  Gain1 : Gain  Gain=c
  Gain2 : Gain  Gain=k
  Math Function : Math  Operator=log
  Product : Product
  Sign : Signum
  Sum : Sum  Inputs=+++
  Sum1 : Sum  Inputs=++|
  Sx : Outport
  wires:
  Gain2/1 -> Sum1/2
  Sign/1 -> Product/1
  Gain1/1 -> Sum/1
  e/1 -> Gain/1, Sign/1, Abs/1
  Math Function/1 -> Product/2
  Sum/1 -> Sx/1
  ev/1 -> Sum/3
  Sum1/1 -> Math Function/1
  Product/1 -> Gain1/1
  Abs/1 -> Gain2/1
  Constant/1 -> Sum1/1
  Gain/1 -> Sum/2

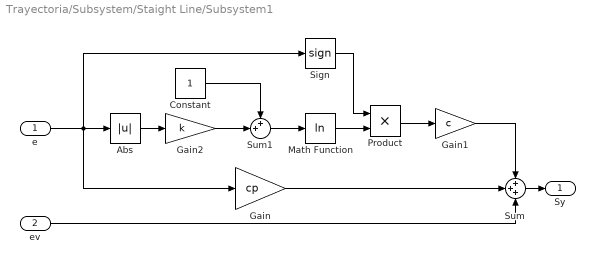
== system Trayectoria/Subsystem/Staight Line/Subsystem1 ==
  e : Inport
  ev : Inport  Port=2
  Abs : Abs  SaturateOnIntegerOverflow=off
  Constant : Constant
  Gain : Gain  Gain=cp
  Gain1 : Gain  Gain=c
  Gain2 : Gain  Gain=k
  Math Function : Math  Operator=log
  Product : Product
  Sign : Signum
  Sum : Sum  Inputs=+++
  Sum1 : Sum  Inputs=++|
  Sy : Outport
  wires:
  Gain/1 -> Sum/2
  Constant/1 -> Sum1/1
  Abs/1 -> Gain2/1
  Product/1 -> Gain1/1
  Sum1/1 -> Math Function/1
  ev/1 -> Sum/3
  Sum/1 -> Sy/1
  Math Function/1 -> Product/2
  e/1 -> Abs/1, Sign/1, Gain/1
  Gain1/1 -> Sum/1
  Sign/1 -> Product/1
  Gain2/1 -> Sum1/2

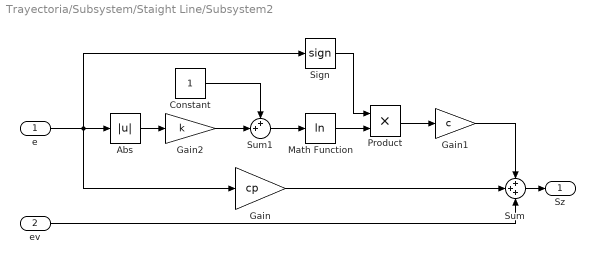
== system Trayectoria/Subsystem/Staight Line/Subsystem2 ==
  e : Inport
  ev : Inport  Port=2
  Abs : Abs  SaturateOnIntegerOverflow=off
  Constant : Constant
  Gain : Gain  Gain=cp
  Gain1 : Gain  Gain=c
  Gain2 : Gain  Gain=k
  Math Function : Math  Operator=log
  Product : Product
  Sign : Signum
  Sum : Sum  Inputs=+++
  Sum1 : Sum  Inputs=++|
  Sz : Outport
  wires:
  Gain2/1 -> Sum1/2
  Sign/1 -> Product/1
  Gain1/1 -> Sum/1
  e/1 -> Gain/1, Sign/1, Abs/1
  Math Function/1 -> Product/2
  Sum/1 -> Sz/1
  ev/1 -> Sum/3
  Sum1/1 -> Math Function/1
  Product/1 -> Gain1/1
  Abs/1 -> Gain2/1
  Constant/1 -> Sum1/1
  Gain/1 -> Sum/2
